simulink model "uav_adrc"  (R2024b)
settings: Solver=FixedStepAuto  StartTime=0.0  StopTime=10.0  FixedStep=0.001  RelTol=1e-3
libraries: slctrl_adaptive x6
settings Model: Creator=nanwan  LastModifiedBy=nanwan
settings OptimizationCC: DefaultParameterBehavior=Inlined  StrengthReduction=on  PassReuseOutputArgsAs=Individual arguments  ZeroExternalMemoryAtStartup=off  ZeroInternalMemoryAtStartup=off  OptimizeBlockOrder=speed  OptimizationPriority=Speed  OptimizationCustomize=off  MultiThreadedLoops=on  AutoScheduleForLoops=on  EfficientTunableParamExpr=on
settings DebuggingCC: ParameterTunabilityLossMsg=error
settings HardwareCC: ProdBitPerLong=64  ProdHWDeviceType=Intel->x86-64 (Linux 64)
settings SFSimCC: MATLABDynamicMemAlloc=off
settings RTWCC: Description=Embedded Coder  SystemTargetFile=ert.tlc  TemplateMakefile=ert_default_tmf  BuildConfiguration=Faster Runs  TargetLang=C++
settings CodeAppCC: ForceParamTrailComments=on  IgnoreCustomStorageClasses=off  OperatorAnnotations=on  SimulinkDataObjDesc=on  SFDataObjDesc=on  InsertBlockDesc=on
settings ERTTargetCC: TargetLangStandard=C++17 (ISO)  GenerateSampleERTMain=on  CodeInterfacePackaging=C++ class  RootIOFormat=Structure reference  ERTCustomFileTemplate=example_file_process.tlc

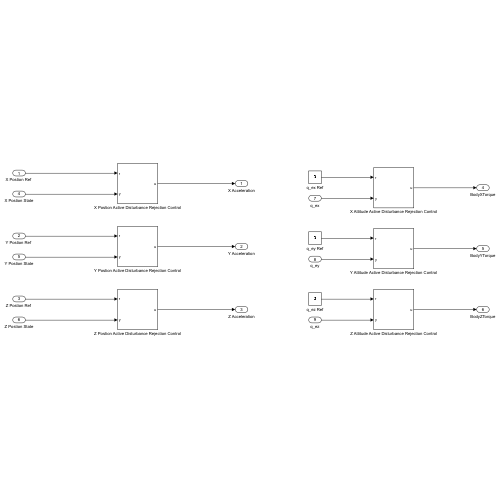
[thumbnail: Simulink's stored preview of the top-level diagram]
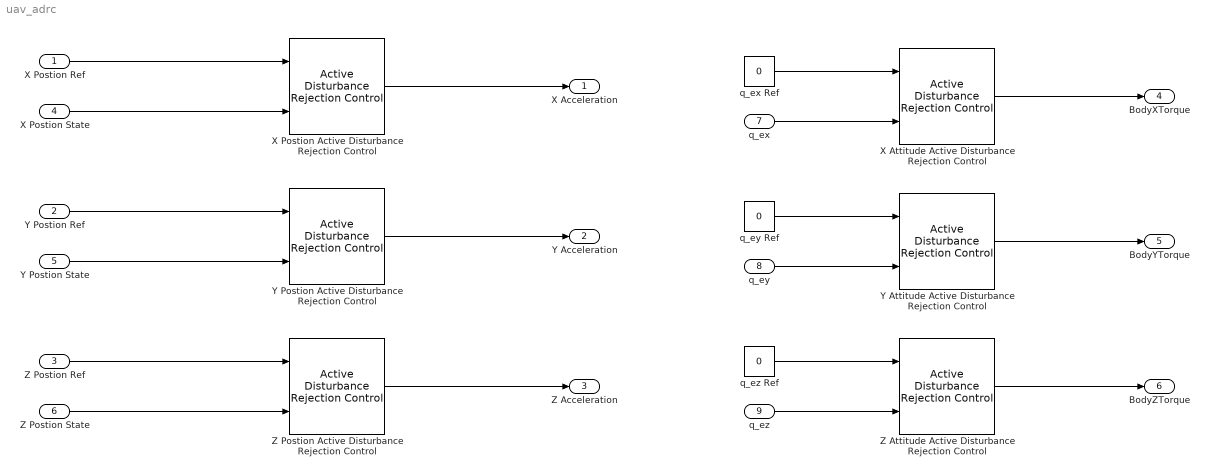
== system uav_adrc ==
  "X Postion Ref " : Inport  OutDataTypeStr=double
  "Y Postion Ref " : Inport  Port=2  OutDataTypeStr=double
  "Z Postion Ref " : Inport  Port=3
  X Postion State : Inport  Port=4  OutDataTypeStr=double
  Y Postion State : Inport  Port=5  OutDataTypeStr=double
  Z Postion State : Inport  Port=6
  q_ex : Inport  Port=7
  q_ey : Inport  Port=8
  q_ez : Inport  Port=9
  X Attitude Active Disturbance Rejection Control : slctrl_adaptive/Active Disturbance Rejection Control  time_domain=discrete-time  Ts=0.001  model_type=second-order  b0=1  wc=1  wo=10  x0=0  ulim_checkbox=off  umax=inf  umin=-inf  xhat_checkbox=off
      settings: LibrarySourceBlock=slctrlblks/Adaptive Control/Active Disturbance Rejection Control
  X Postion Active Disturbance Rejection Control : slctrl_adaptive/Active Disturbance Rejection Control  time_domain=discrete-time  Ts=0.001  model_type=second-order  b0=1  wc=1  wo=10  x0=0  ulim_checkbox=off  umax=inf  umin=-inf  xhat_checkbox=off
      settings: LibrarySourceBlock=slctrlblks/Adaptive Control/Active Disturbance Rejection Control
  Y Attitude Active Disturbance Rejection Control : slctrl_adaptive/Active Disturbance Rejection Control  time_domain=discrete-time  Ts=0.001  model_type=second-order  b0=1  wc=1  wo=10  x0=0  ulim_checkbox=off  umax=inf  umin=-inf  xhat_checkbox=off
      settings: LibrarySourceBlock=slctrlblks/Adaptive Control/Active Disturbance Rejection Control
  Y Postion Active Disturbance Rejection Control : slctrl_adaptive/Active Disturbance Rejection Control  time_domain=discrete-time  Ts=0.001  model_type=second-order  b0=1  wc=1  wo=10  x0=0  ulim_checkbox=off  umax=inf  umin=-inf  xhat_checkbox=off
      settings: LibrarySourceBlock=slctrlblks/Adaptive Control/Active Disturbance Rejection Control
  Z Attitude Active Disturbance Rejection Control : slctrl_adaptive/Active Disturbance Rejection Control  time_domain=discrete-time  Ts=0.001  model_type=second-order  b0=1  wc=1  wo=10  x0=0  ulim_checkbox=off  umax=inf  umin=-inf  xhat_checkbox=off
      settings: LibrarySourceBlock=slctrlblks/Adaptive Control/Active Disturbance Rejection Control
  Z Postion Active Disturbance Rejection Control : slctrl_adaptive/Active Disturbance Rejection Control  time_domain=discrete-time  Ts=0.001  model_type=second-order  b0=1  wc=1  wo=10  x0=0  ulim_checkbox=off  umax=inf  umin=-inf  xhat_checkbox=off
      settings: LibrarySourceBlock=slctrlblks/Adaptive Control/Active Disturbance Rejection Control
  q_ex Ref : Constant  Value=0
  q_ey Ref : Constant  Value=0
  q_ez Ref : Constant  Value=0
  X Acceleration : Outport
  Y Acceleration : Outport  Port=2
  Z Acceleration : Outport  Port=3
  BodyXTorque : Outport  Port=4
  BodyYTorque : Outport  Port=5
  BodyZTorque : Outport  Port=6
  wires:
  "X Postion Ref "/1 -> X Postion Active Disturbance Rejection Control/1
  "Y Postion Ref "/1 -> Y Postion Active Disturbance Rejection Control/1
  "Z Postion Ref "/1 -> Z Postion Active Disturbance Rejection Control/1
  X Postion State/1 -> X Postion Active Disturbance Rejection Control/2
  Y Postion State/1 -> Y Postion Active Disturbance Rejection Control/2
  Z Postion State/1 -> Z Postion Active Disturbance Rejection Control/2
  X Postion Active Disturbance Rejection Control/1 -> X Acceleration/1
  Y Postion Active Disturbance Rejection Control/1 -> Y Acceleration/1
  Z Postion Active Disturbance Rejection Control/1 -> Z Acceleration/1
  q_ex Ref/1 -> X Attitude Active Disturbance Rejection Control/1
  q_ey Ref/1 -> Y Attitude Active Disturbance Rejection Control/1
  q_ez Ref/1 -> Z Attitude Active Disturbance Rejection Control/1
  q_ex/1 -> X Attitude Active Disturbance Rejection Control/2
  q_ey/1 -> Y Attitude Active Disturbance Rejection Control/2
  q_ez/1 -> Z Attitude Active Disturbance Rejection Control/2
  X Attitude Active Disturbance Rejection Control/1 -> BodyXTorque/1
  Z Attitude Active Disturbance Rejection Control/1 -> BodyZTorque/1
  Y Attitude Active Disturbance Rejection Control/1 -> BodyYTorque/1
